simulink model "drive_test"  (R2016a)
settings: Solver=VariableStepAuto  StartTime=0.0  StopTime=10.0  FixedStep=0.001  RelTol=1e-3
settings Model: Creator=maximilian  LastModifiedBy=maximilian

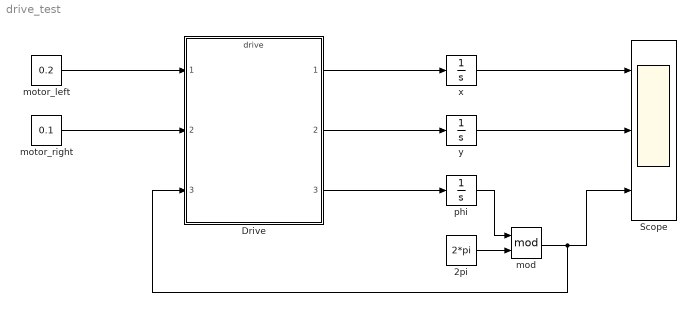
== system drive_test ==
  2pi : Constant  Value=2*pi
  Drive : ModelReference  ModelNameDialog=drive.mdl  SimulationMode=Normal  ModelReferenceVersion=1.12
  Scope : Scope  NumInputPorts=3
  mod : Math  Operator=mod  SaturateOnIntegerOverflow=on
  motor_left : Constant  Value=0.2
  motor_right : Constant  Value=0.1
  phi : Integrator
  x : Integrator
  y : Integrator
  wires:
  Drive/1 -> x/1
  motor_left/1 -> Drive/1
  motor_right/1 -> Drive/2
  x/1 -> Scope/1
  Drive/2 -> y/1
  Drive/3 -> phi/1
  y/1 -> Scope/2
  phi/1 -> mod/1
  mod/1 -> Drive/3, Scope/3
  2pi/1 -> mod/2
